simulink model "ESP32Arm5DOF(conflicted copy 04-16-2025 11_18_05)"  (R2024a)
settings: Solver=VariableStepAuto  StartTime=0.0  StopTime=10.0  RelTol=1e-3
libraries: SignalEditorBlockLib x5, arduinolib x5, arduinosensorlib x1
settings Model: Creator=Akbar  LastModifiedBy=Akbar

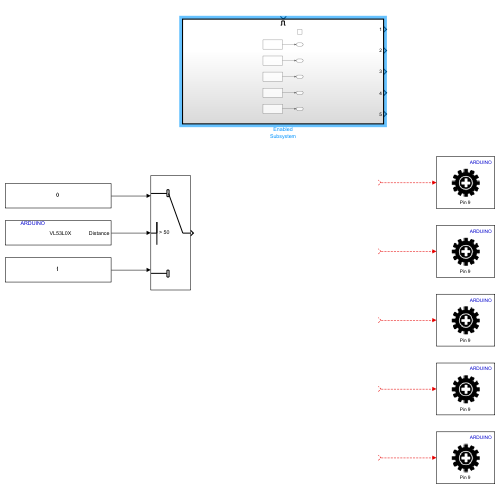
[thumbnail: Simulink's stored preview of the top-level diagram]
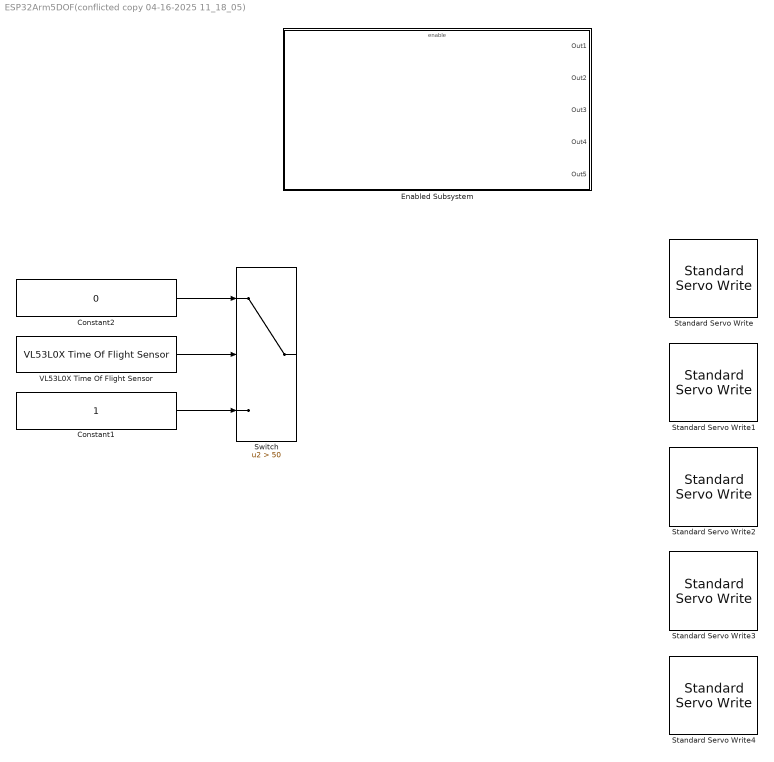
== system ESP32Arm5DOF(conflicted copy 04-16-2025 11_18_05) ==
  Constant1 : Constant
  Constant2 : Constant  Value=0
  Enabled Subsystem : Subsystem  TreatAsAtomicUnit=on
  Standard Servo Write{,1..4} (5 alike) : arduinolib/Standard Servo Write  pinNumber=9  ServoIndex=0  blockPlatform=ARDUINO
  Switch : Switch  Criteria=u2 > Threshold  Threshold=50  SaturateOnIntegerOverflow=off  InputSameDT=off
  VL53L0X Time Of Flight Sensor : arduinosensorlib/VL53L0X Time Of Flight Sensor  I2CModule=0  I2CAddress=0x29  BitRate=1000000  RangingMode=Default  SampleTime=-1
  wires:
  VL53L0X Time Of Flight Sensor/1 -> Switch/2
  Constant2/1 -> Switch/1
  Constant1/1 -> Switch/3
  ? -> Standard Servo Write2/1
  ? -> Standard Servo Write4/1
  ? -> Standard Servo Write/1
  ? -> Standard Servo Write3/1
  ? -> Standard Servo Write1/1

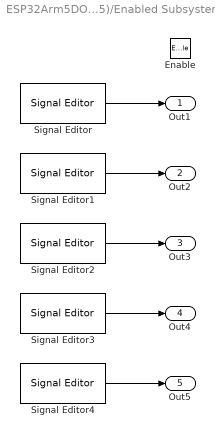
== system ESP32Arm5DOF(conflicted copy 04-16-2025 11_18_05)/Enabled Subsystem ==
  Enable : EnablePort
  Signal Editor{,1..4} (5 alike) : SignalEditorBlockLib/Signal Editor  FileName=untitled.mat  ActiveScenario=Scenario  ActiveSignal=Signal 1  IsBus=off  OutputBusObjectStr=Bus: BusObject  SampleTime=0  Interpolate=off  ZeroCross=off  OutputAfterFinalValue=Setting to zero  Unit=inherit  PreserveSignalName=on  ApplySigPropsToAllScenarios=on  ApplySigPropsToAllSignals=off
  Out1 : Outport
  Out2 : Outport  Port=2
  Out3 : Outport  Port=3
  Out4 : Outport  Port=4
  Out5 : Outport  Port=5
  wires:
  Signal Editor/1 -> Out1/1
  Signal Editor1/1 -> Out2/1
  Signal Editor2/1 -> Out3/1
  Signal Editor3/1 -> Out4/1
  Signal Editor4/1 -> Out5/1
